simulink model "Initial_Data"  (R2021b)
settings: Solver=VariableStepAuto  StartTime=0.0  StopTime=inf  RelTol=1e-3
libraries: slrealtimeutilitieslib x1, dspnetwork x1
settings Model: Creator=dmgp1  LastModifiedBy=dmgp1

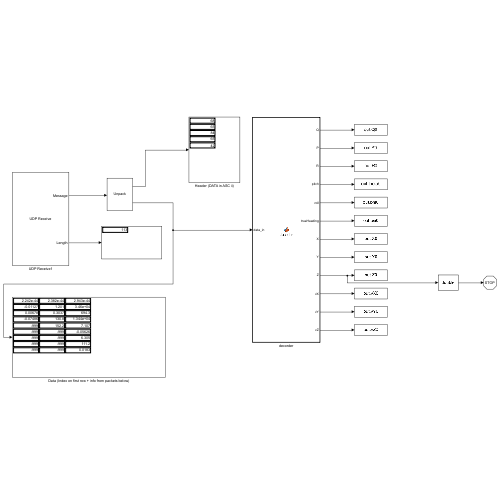
[thumbnail: Simulink's stored preview of the top-level diagram]
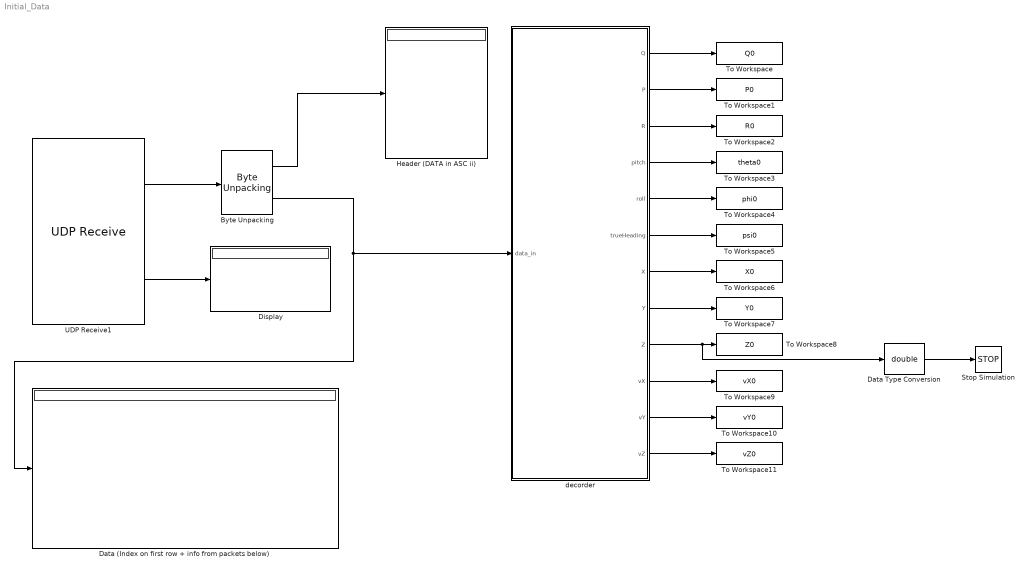
== system Initial_Data ==
  Byte Unpacking : slrealtimeutilitieslib/Byte Unpacking  MaskUnpackedDataTypes={'uint8','single'}  MaskUnpackedDataSizes={5,[9,3]}  MaskAlignment=1
      settings: SourceProductBaseCode=XP
  Data (Index on first row + info from packets below) : Display
  Data Type Conversion : DataTypeConversion  OutDataTypeStr=double
  Display : Display
  Header (DATA in ASC ii) : Display
  Stop Simulation : Stop
  To Workspace : ToWorkspace  VariableName=Q0  SampleTime=-1
      settings: Save2DSignal=2-D array (concatenate along first dimension)
  To Workspace1 : ToWorkspace  VariableName=P0  SampleTime=-1
      settings: Save2DSignal=2-D array (concatenate along first dimension)
  To Workspace10 : ToWorkspace  VariableName=vY0  SampleTime=-1
      settings: Save2DSignal=2-D array (concatenate along first dimension)
  To Workspace11 : ToWorkspace  VariableName=vZ0  SampleTime=-1
      settings: Save2DSignal=2-D array (concatenate along first dimension)
  To Workspace2 : ToWorkspace  VariableName=R0  SampleTime=-1
      settings: Save2DSignal=2-D array (concatenate along first dimension)
  To Workspace3 : ToWorkspace  VariableName=theta0  SampleTime=-1
      settings: Save2DSignal=2-D array (concatenate along first dimension)
  To Workspace4 : ToWorkspace  VariableName=phi0  SampleTime=-1
      settings: Save2DSignal=2-D array (concatenate along first dimension)
  To Workspace5 : ToWorkspace  VariableName=psi0  SampleTime=-1
      settings: Save2DSignal=2-D array (concatenate along first dimension)
  To Workspace6 : ToWorkspace  VariableName=X0  SampleTime=-1
      settings: Save2DSignal=2-D array (concatenate along first dimension)
  To Workspace7 : ToWorkspace  VariableName=Y0  SampleTime=-1
      settings: Save2DSignal=2-D array (concatenate along first dimension)
  To Workspace8 : ToWorkspace  VariableName=Z0  SampleTime=-1
      settings: Save2DSignal=2-D array (concatenate along first dimension)
  To Workspace9 : ToWorkspace  VariableName=vX0  SampleTime=-1
      settings: Save2DSignal=2-D array (concatenate along first dimension)
  UDP Receive1 : dspnetwork/UDP Receive  localURL='0.0.0.0'  localPort=49004  remoteURL='127.0.0.1'  remotePort=-1  recvBufferSize=8192  dims=113  signalDatatype=uint8  isComplex=off  isVarSize=off  showBlockingTime=off  blockingTime=0  sampletime=inf  blockPlatform=[]
  decorder : MATLAB Function  TreatAsAtomicUnit=on
  wires:
  UDP Receive1/2 -> Display/1
  UDP Receive1/1 -> Byte Unpacking/1
  Byte Unpacking/1 -> Header (DATA in ASC ii)/1
  Byte Unpacking/2 -> Data (Index on first row + info from packets below)/1, decorder/1(data_in)
  decorder/1(Q) -> To Workspace/1
  decorder/2(P) -> To Workspace1/1
  decorder/3(R) -> To Workspace2/1
  decorder/4(pitch) -> To Workspace3/1
  decorder/5(roll) -> To Workspace4/1
  decorder/7(X) -> To Workspace6/1
  decorder/8(Y) -> To Workspace7/1
  decorder/6(trueHeading) -> To Workspace5/1
  decorder/9(Z) -> Data Type Conversion/1, To Workspace8/1
  Data Type Conversion/1 -> Stop Simulation/1
  decorder/10(vX) -> To Workspace9/1
  decorder/11(vY) -> To Workspace10/1
  decorder/12(vZ) -> To Workspace11/1

== matlab function Initial_Data/decorder ==
  data: data_in input; Q output; P output; R output; pitch output; roll output; trueHeading output; X output; Y output; Z output; vX output; vY output; vZ output
function [Q, P, R, pitch,roll, trueHeading, X,Y,Z,vX,vY,vZ] = decoder(data_in)

% Remember that the first item in each column is the index converted to single (useless)

Q = data_in(2,1);
P = data_in(3,1);
R = data_in(4,1);

pitch = data_in(2,2);
roll = data_in(3,2);
trueHeading = data_in(4,2); 

X = data_in(2,3);
Y = data_in(3,3);
Z = data_in(4,3);

vX = data_in(5,3);
vY = data_in(6,3);
vZ = data_in(7,3);

end
